simulink model "part3"  (R2024b)
settings: Solver=VariableStepAuto  StartTime=0.0  StopTime=0.2  RelTol=1e-3
undefined symbols (not defined in the file): f, U_out
libraries: cstblocks x4
settings Model: Creator=Andrei  LastModifiedBy=Andrei

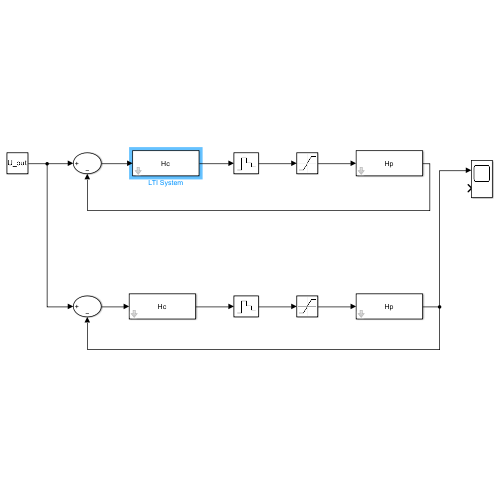
[thumbnail: Simulink's stored preview of the top-level diagram]
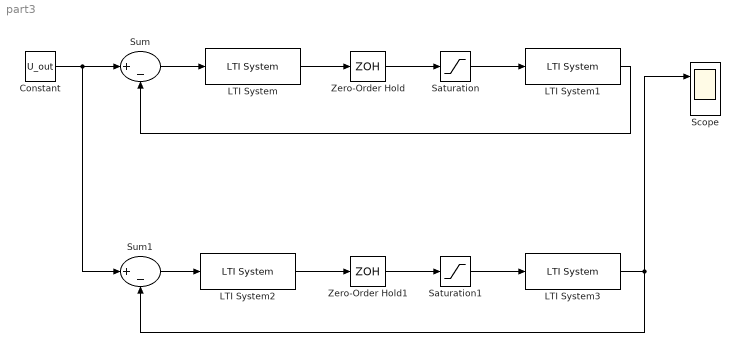
== system part3 ==
  Constant : Constant  Value=U_out
  LTI System : cstblocks/LTI System  sys=Hc  IC=[]  PadeOrder=0
  LTI System1 : cstblocks/LTI System  sys=Hp  IC=[]  PadeOrder=0
  LTI System2 : cstblocks/LTI System  sys=Hc  IC=[]  PadeOrder=0
  LTI System3 : cstblocks/LTI System  sys=Hp  IC=[]  PadeOrder=0
  Saturation : Saturate  UpperLimit=1  LowerLimit=0
  Saturation1 : Saturate  UpperLimit=1  LowerLimit=0
  Scope : Scope  NumInputPorts=2
  Sum : Sum  Inputs=|+-
  Sum1 : Sum  Inputs=|+-
  Zero-Order Hold : ZeroOrderHold  SampleTime=1/f/10
  Zero-Order Hold1 : ZeroOrderHold  SampleTime=1/f
  wires:
  LTI System1/1 -> Sum/2
  Saturation/1 -> LTI System1/1
  Zero-Order Hold/1 -> Saturation/1
  LTI System/1 -> Zero-Order Hold/1
  Sum/1 -> LTI System/1
  LTI System2/1 -> Zero-Order Hold1/1
  Constant/1 -> Sum1/1, Sum/1
  LTI System3/1 -> Scope/1, Sum1/2
  Zero-Order Hold1/1 -> Saturation1/1
  Sum1/1 -> LTI System2/1
  Saturation1/1 -> LTI System3/1
